simulink model "fig10_81_Ecoli"  (Simulink 7.0)
settings: Solver=ode45  StartTime=0.0  StopTime=40.0  RelTol=1e-3
settings Model: Creator=Gene Franklin  LastModifiedBy=abbas
settings DebuggingCC: SaveWithParameterizedLinksMsg=none
settings GRTTargetCC: TargetFcnLib=ansi_tfl_tmw.mat

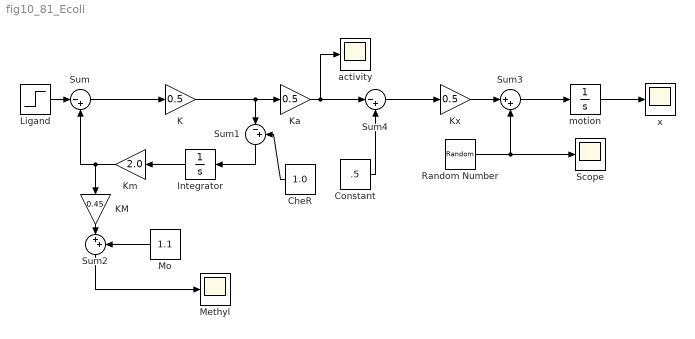
== system fig10_81_Ecoli ==
  CheR : Constant  Orientation=left  Value=1.0  OutDataType=sfix(16)  OutScaling=2^0
  Constant : Constant  Value=.5  OutDataType=sfix(16)  OutScaling=2^0
  Integrator : Integrator  Orientation=left  InitialCondition=1.0
  K : Gain  Gain=0.5  ParameterDataType=sfix(16)  ParameterScaling=2^0  OutDataType=sfix(16)  OutScaling=2^0
  KM : Gain  Orientation=down  Gain=0.45  ParameterDataType=sfix(16)  ParameterScaling=2^0  OutDataType=sfix(16)  OutScaling=2^0
  Ka : Gain  Gain=0.5  ParameterDataType=sfix(16)  ParameterScaling=2^0  OutDataType=sfix(16)  OutScaling=2^0
  Km : Gain  Orientation=left  Gain=2.0  ParameterDataType=sfix(16)  ParameterScaling=2^0  OutDataType=sfix(16)  OutScaling=2^0
  Kx : Gain  Gain=0.5  ParameterDataType=sfix(16)  ParameterScaling=2^0  OutDataType=sfix(16)  OutScaling=2^0
  Ligand : Step  Time=20  After=2.0  SampleTime=0
  Methyl : Scope
      settings: SaveName=EcoliMeth  DataFormat=Array
  Mo : Constant  Orientation=left  Value=1.1  OutDataType=sfix(16)  OutScaling=2^0
  Random Number : RandomNumber  Variance=0.002  SampleTime=0.5
  Scope : Scope
  Sum : Sum  Inputs=|-+  OutDataType=sfix(16)  OutScaling=2^0
  Sum1 : Sum  Orientation=down  Inputs=|-+  OutDataType=sfix(16)  OutScaling=2^0
  Sum2 : Sum  Orientation=down  Inputs=|++  OutDataType=sfix(16)  OutScaling=2^0
  Sum3 : Sum  Inputs=|++  OutDataType=sfix(16)  OutScaling=2^0
  Sum4 : Sum  Inputs=|-+  OutDataType=sfix(16)  OutScaling=2^0
  activity : Scope
      settings: SaveName=EcoliA  DataFormat=Array
  motion : Integrator
  x : Scope
      settings: SaveName=Ecolix  DataFormat=Array
  wires:
  Ligand/1 -> Sum/1
  Sum/1 -> K/1
  Integrator/1 -> Km/1
  Sum1/1 -> Integrator/1
  CheR/1 -> Sum1/2
  K/1 -> Sum1/1, Ka/1
  Km/1 -> Sum/2, KM/1
  Mo/1 -> Sum2/2
  KM/1 -> Sum2/1
  Sum2/1 -> Methyl/1
  motion/1 -> x/1
  Kx/1 -> Sum3/1
  Sum3/1 -> motion/1
  Ka/1 -> Sum4/1, activity/1
  Sum4/1 -> Kx/1
  Constant/1 -> Sum4/2
  Random Number/1 -> Sum3/2, Scope/1
